simulink library "GS_refuel_control_R2024a"  (R2024a)
settings: Solver=VariableStepAuto  StartTime=0.0  StopTime=10.0  RelTol=1e-3
undefined symbols (not defined in the file or in its folder): ABORT_MODE, CHILLDOWN, CLOSE, CONNECTED, DEFUEL, DISCONNECTED, IDLE, OPEN, REFUEL, timestep, WARMUP
settings Model: Creator=MW  LastModifiedBy=MW

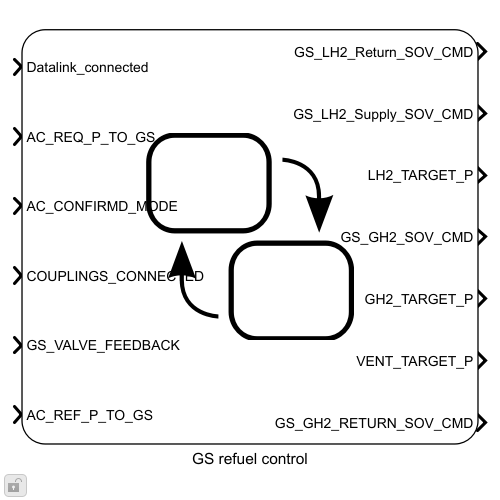
[thumbnail: Simulink's stored preview of the top-level diagram]
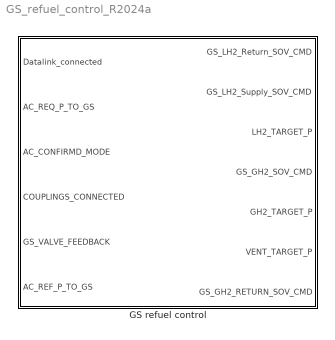
== system GS_refuel_control_R2024a ==
  GS refuel control : Stateflow chart  TreatAsAtomicUnit=on  SystemSampleTime=timestep

== stateflow chart GS_refuel_control_R2024a/GS refuel control ==
  state IDLE
    en:
    GS_LH2_Supply_SOV_CMD = CLOSE;
    GS_LH2_Return_SOV_CMD = CLOSE;
    LH2_TARGET_P = IDLE_P;
    GH2_TARGET_P = IDLE_P;
    VENT_TARGET_P = IDLE_P;
    GS_GH2_SOV_CMD = OPEN;
    GS_GH2_RETURN_SOV_CMD = OPEN;
  state EMERGENCY_STOP
    en:
    GS_LH2_Supply_SOV_CMD = CLOSE;
    GS_LH2_Return_SOV_CMD = CLOSE;
    GS_GH2_SOV_CMD = CLOSE;
  state CHECK_INTEGRITY
    en:
    GS_LH2_Supply_SOV_CMD = CLOSE;
    GS_LH2_Return_SOV_CMD = CLOSE;
    GS_GH2_SOV_CMD = OPEN;
    GS_GH2_RETURN_SOV_CMD = OPEN;
  state CHILLDOWN
    en, du:
    GH2_TARGET_P =  IDLE_P;
    VENT_TARGET_P = min(MAX_P, AC_REF_P_TO_GS);
    LH2_TARGET_P = min(MAX_P, AC_REQ_P_TO_GS);
    GS_LH2_Supply_SOV_CMD = OPEN;
    GS_LH2_Return_SOV_CMD = OPEN;
    GS_GH2_SOV_CMD = CLOSE;
    GS_GH2_RETURN_SOV_CMD = CLOSE;
  state TANK_FILL
    en, du:
    GH2_TARGET_P =  IDLE_P;
    VENT_TARGET_P = min(MAX_P, AC_REF_P_TO_GS);
    LH2_TARGET_P = min(MAX_P, AC_REQ_P_TO_GS);
    GS_LH2_Supply_SOV_CMD = OPEN;
    GS_LH2_Return_SOV_CMD = OPEN;
    GS_GH2_SOV_CMD = CLOSE;
    GS_GH2_RETURN_SOV_CMD = CLOSE;
  state TANK_DRAIN
    en, du:
    VENT_TARGET_P = min(MAX_P, AC_REF_P_TO_GS);
    GH2_TARGET_P = min(MAX_P, AC_REQ_P_TO_GS);
    LH2_TARGET_P = IDLE_P;
    GS_LH2_Supply_SOV_CMD = CLOSE;
    GS_LH2_Return_SOV_CMD = CLOSE;
    GS_GH2_SOV_CMD = OPEN;
    GS_GH2_RETURN_SOV_CMD = OPEN;
  state WARMUP
    en, du:
    VENT_TARGET_P = min(MAX_P, AC_REF_P_TO_GS);
    LH2_TARGET_P =  IDLE_P;
    GH2_TARGET_P = min(MAX_P, AC_REQ_P_TO_GS);
    GS_LH2_Supply_SOV_CMD = CLOSE;
    GS_LH2_Return_SOV_CMD = CLOSE;
    GS_GH2_SOV_CMD = OPEN;
    GS_GH2_RETURN_SOV_CMD = OPEN;
  state DISCONNECT
    en:
    VENT_TARGET_P = IDLE_P;
    LH2_TARGET_P =  IDLE_P;
    GH2_TARGET_P = IDLE_P;
    GS_LH2_Supply_SOV_CMD = CLOSE;
    GS_LH2_Return_SOV_CMD = CLOSE;
    GS_GH2_SOV_CMD = OPEN;
    GS_GH2_RETURN_SOV_CMD = OPEN;
  (default) -> IDLE
  IDLE -> EMERGENCY_STOP [order 1] : [AC_CONFIRMD_MODE == ABORT_MODE]
  DISCONNECT -> IDLE [order 2] : [COUPLINGS_CONNECTED == DISCONNECTED && ...
      | Datalink_connected == DISCONNECTED]
  IDLE -> CHECK_INTEGRITY [order 2] : [Datalink_connected == CONNECTED]
  CHECK_INTEGRITY -> EMERGENCY_STOP [order 1] : [AC_CONFIRMD_MODE == ABORT_MODE]
  CHECK_INTEGRITY -> CHILLDOWN [order 2] : [AC_CONFIRMD_MODE == CHILLDOWN && ...
      | COUPLINGS_CONNECTED == CONNECTED]
  CHILLDOWN -> EMERGENCY_STOP [order 1] : [AC_CONFIRMD_MODE == ABORT_MODE]
  CHILLDOWN -> TANK_DRAIN [order 3] : [AC_CONFIRMD_MODE == DEFUEL]
  CHILLDOWN -> TANK_FILL [order 2] : [AC_CONFIRMD_MODE == REFUEL]
  TANK_FILL -> EMERGENCY_STOP [order 1] : [AC_CONFIRMD_MODE == ABORT_MODE]
  TANK_FILL -> WARMUP [order 2] : [AC_CONFIRMD_MODE == WARMUP]
  TANK_DRAIN -> EMERGENCY_STOP [order 1] : [AC_CONFIRMD_MODE == ABORT_MODE]
  TANK_DRAIN -> DISCONNECT [order 2] : [AC_CONFIRMD_MODE == IDLE]
  WARMUP -> EMERGENCY_STOP [order 1] : [AC_CONFIRMD_MODE == ABORT_MODE]
  WARMUP -> DISCONNECT [order 2] : [AC_CONFIRMD_MODE == IDLE]
  DISCONNECT -> EMERGENCY_STOP [order 1] : [AC_CONFIRMD_MODE == ABORT_MODE]
  data: Datalink_connected input; GS_LH2_Return_SOV_CMD output; GS_LH2_Supply_SOV_CMD output; CLOSE parameter; OPEN parameter; AC_REQ_P_TO_GS input; LH2_TARGET_P output double; AC_CONFIRMD_MODE input; CHILLDOWN parameter; DEFUEL parameter; IDLE parameter; REFUEL parameter; WARMUP parameter; COUPLINGS_CONNECTED input; CONNECTED parameter; DISCONNECTED parameter; GS_GH2_SOV_CMD output; GH2_TARGET_P output double; ABORT_MODE parameter; MAX_P constant double =0.5; IDLE_P constant double =0.12; VENT_TARGET_P output; GS_VALVE_FEEDBACK input Bus: GS_VALVE_FEEDBACK; AC_REF_P_TO_GS input; GS_GH2_RETURN_SOV_CMD output
